simulink model "F2837x_CPU1_bissc"  (R2020b)
settings: Solver=FixedStepDiscrete  StartTime=0.0  StopTime=Inf  FixedStep=0.2  RelTol=1e-3  EnableMultiTasking=on
undefined symbols (not defined in the file): BISS_DATA_CLOCKS, BISS_POSITION_BITS, BISS_POSITION_CRC_BITS, bissc_receivePosition, C28x, CPU1, CPU2, DELAY_US, PM_bissc_setupNewSCDTransfer, PM_bissc_startOperation, SPI_FIFO_WIDTH
libraries: demo_controls x1, c2837xDlib x1, idelinklib_common x1
settings Model: ExtModeTrigDuration=8  Creator=vchilapu  LastModifiedBy=User
settings DataIOCC: ReturnWorkspaceOutputs=off
settings OptimizationCC: DefaultUnderspecifiedDataType=single  EnhancedBackFolding=on  PassReuseOutputArgsAs=Individual arguments  MaxStackSize=512  OptimizeBlockOrder=speed  DifferentSizesBufferReuse=on  OptimizationCustomize=off  EfficientTunableParamExpr=on
settings DebuggingCC: ParameterTunabilityLossMsg=error  ArithmeticOperatorsInVariantConditions=warning
settings HardwareCC: ProdBitPerChar=16  ProdBitPerInt=16  ProdBitPerPointer=32  ProdBitPerSizeT=32  ProdBitPerPtrDiffT=32  ProdLargestAtomicInteger=Integer  ProdLargestAtomicFloat=None  ProdWordSize=16  ProdLongLongMode=on  ProdHWDeviceType=Texas Instruments->C2000
settings SFSimCC: MATLABDynamicMemAlloc=off  CustomCodeUndefinedFunction=UseInterfaceOnly
settings RTWCC: Description=Embedded Coder  SystemTargetFile=ert.tlc  HardwareBoard=TI Delfino F28379D LaunchPad  TemplateMakefile=ert_default_tmf  GenerateReport=on  CustomHeaderCode="#include \"bissc.h\""  CustomSource=bissc.c  CustomLibrary=PM_bissC_Lib.lib  Toolchain=Texas Instruments Code Composer Studio (C2000)  IncludeHyperlinkInReport=on  LaunchReport=on  GenerateTraceInfo=on  GenerateTraceReport=on  GenerateTraceReportSl=on  GenerateTraceReportSf=on  GenerateTraceReportEml=on
settings RTWCC: CustomInclude=|
  | C:/ti/controlSUITE/development_kits/BOOSTXL_POSMGR/v01_01_00_00/bissc-F28379DLpad-S2/examples/PM_bissc_SystemTest/
  | C:/ti/controlSUITE/development_kits/BOOSTXL_POSMGR/v01_01_00_00/bissc-F28379DLpad-S2/Float/include/
  | C:\ti\controlSUITE\development_kits\BOOSTXL_POSMGR\v01_01_00_00\bissc-F28379DLpad-S2\Float\lib
settings CodeAppCC: ForceParamTrailComments=on  IgnoreCustomStorageClasses=off  OperatorAnnotations=on  SimulinkDataObjDesc=on  SFDataObjDesc=on  InsertBlockDesc=on
settings ERTTargetCC: CodeReplacementLibrary=TI C28x

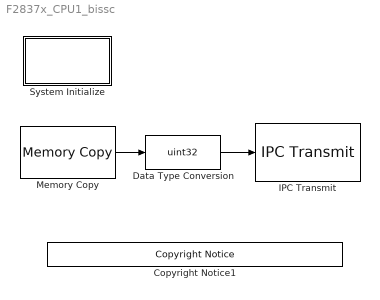
== system F2837x_CPU1_bissc ==
  Copyright Notice1 : demo_controls/Copyright Notice  year=2021  prod=tic2000
      settings: SourceProductBaseCode=ME
  Data Type Conversion : DataTypeConversion  OutDataTypeStr=uint32
  IPC Transmit : c2837xDlib/IPC Transmit  blkParamProc=F2837x  SelectDestination=C28x (CPU1/CPU2)  SelectChannel=0  EnableBlocking=off
      settings: SourceProductBaseCode=TIC2000
  Memory Copy : idelinklib_common/Memory Copy  copyFrom=Specified source code symbol  copyFromAddressSource=Specify via dialog  copyFromAddress=hex2dec('00001000')  copyFromSrcCode=&bissc_data_struct.position  dataTypeFrom=uint32  dataDimensionFrom=1  useOffsetFrom=off  offsetFromSrc=Specify via dialog  offsetFrom=0  strideFrom=1  copyTo=Output port  copyToAddressSource=Specify via dialog  copyToAddress=hex2dec('00002000')  copyToSrcCode=myVariableDst  dataTypeTo=uint32  useOffsetTo=off  offsetToSrc=Specify via dialog  offsetTo=0  strideTo=1  sampleTime=-1  useInitValue=off  initValueSrc=Specify constant value  initValue=1  initValueSrcCode=myInitValueVariable  useAsMask=off  maskOperator=bitwise AND  useTermValue=off  termValue=1  isRealtimeEnabled=off  emitCCBeforeWrite=on  CCBeforeWrite=PM_bissc_setupNewSCDTransfer(BISS_DATA_CLOCKS, SPI_FIFO_WIDTH); DELAY_US(10L);PM_bissc_startOperation();bissc_receivePosition(BISS_POSITION_BITS, BISS_POSITION_CRC_BITS) ;  emitCCAfterWrite=off  CCAfterWrite=/* Custom Code After Write*/  useDMACopy=off  enableBlockingMode=off
      settings: SourceProductBaseCode=ME
  System Initialize : Subsystem  mask(System Initialize){ShowInLibBrowser=0}
      mask prompts: ShowInLibBrowser "Simulink:masks:CustCodeMaskParam1_MP"
      settings: CopyFcn=cccopyfcn(gcb)  OpenFcn=ccopenfcn('System Initialize Function')
      mask Help: eval('feval(''rtwprivate'',''rtwhelpview'',''rtw_sys_initialize_block'')');
      mask Display: disp('System\nInitialize');
  wires:
  Memory Copy/1 -> Data Type Conversion/1
  Data Type Conversion/1 -> IPC Transmit/1

== system F2837x_CPU1_bissc/System Initialize ==
